simulink model "MicrogridDynamics"  (R2020b)
settings: Solver=ode23t  StartTime=0.0  StopTime=1  RelTol=1e-3
values from neighbouring files (symbols this model uses):
  C = 10e-6    (= 1e-05)    [ControllerDesign.m]
  Frq = 50    [ControllerDesign.m]
  Lg = 1.5e-3    (= 0.0015)    [ControllerDesign.m]
  Li = 3e-3    (= 0.003)    [ControllerDesign.m]
  Ll = 10e-3    (= 0.01)    [ControllerDesign.m]
  Rl = 1    [ControllerDesign.m]
  Rld = 50    [ControllerDesign.m]
  Rld1 = 200    [ControllerDesign.m]
  sw_fr = 10e3    (= 10000)    [ControllerDesign.m]
  Vac = 220    [ControllerDesign.m]
  Vdc = 500    [ControllerDesign.m]
undefined symbols (not defined in the file or in its folder): C_pi, C_pi1
libraries: powerlib x61, powerlib_meascontrol x12, pid_lib x8, eeRmsMeasurement x4, eePowerMeasurement x2
(part 1 of 2)
settings Model: Creator=dipsb  LastModifiedBy=dipsb
settings SolverCC: ZeroCrossAlgorithm=Adaptive
settings DebuggingCC: IgnoredZcDiagnostic=none

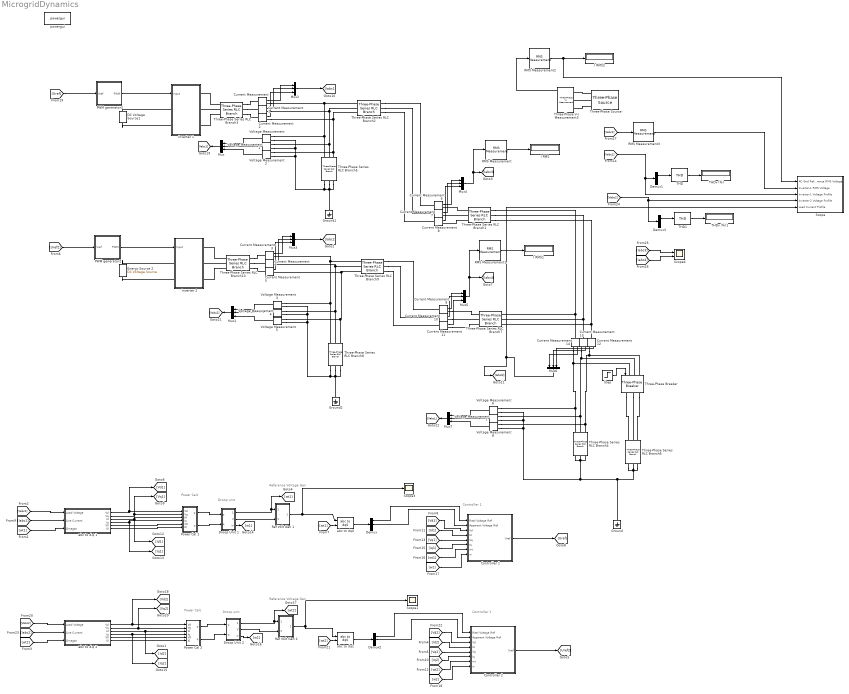
== system MicrogridDynamics ==
  note: Droop unit
  note: Reference Voltage Gen
  note: Reference Voltage Gen
  note: Droop unit
  note: Power Calc
  note: Power Calc
  note: Controller 1
  note: Controller 1
  Controller 1 : Subsystem
  Controller 2 : Subsystem
  Current Measurement{,1..14} (15 alike) : powerlib/Measurements/Current Measurement  PhasorSimulation=off  OutputType=Complex  PSBequivalent=0
  DC Voltage Source1 : powerlib/Electrical Sources/DC Voltage Source  Amplitude=Vdc  Measurements=Voltage
  Demux{,1..3} (4 alike) : Demux  Outputs=3
  Droop Unit 1 : Subsystem
  Droop Unit 2 : Subsystem
  Energy Source 2 : powerlib/Electrical Sources/DC Voltage Source  Amplitude=Vdc  Measurements=Voltage
  Ground : powerlib/Elements/Ground  LConnTagsString=a
  Ground1 : powerlib/Elements/Ground  LConnTagsString=a
  Ground2 : powerlib/Elements/Ground  LConnTagsString=a
  I RMS : Display
  I RMS1 : Display
  I RMS2 : Display
  Inverter 1 : Subsystem
  Inverter 2 : Subsystem
  Mux{,1..7} (8 alike) : Mux  Inputs=3
  PWM generator1 : Subsystem  mask{f=sw_fr}
      mask prompts: f "Frequency (Hz)"
  PWM generator2 : Subsystem  mask{f=sw_fr}
      mask prompts: f "Frequency (Hz)"
  Power Cal 1 : Subsystem
  Power Cal 2 : Subsystem
  RMS Measurement{,1..3} (4 alike) : eeRmsMeasurement/RMS Measurement  LabelModeActiveChoice=Total  F=50  SpecifyHarmonics=off  K=[0 1 2]  Ts=0
      settings: SourceProductBaseCode=PS
  Ref Volt Gen 1 : Subsystem
  Ref Volt Gen 2 : Subsystem
  Scope : Subsystem
  Scope1 : Scope
  Scope3 : Scope
  Scope4 : Scope  NumInputPorts=2
  Step : Step  Time=0.4  SampleTime=0
  THD : powerlib_meascontrol/Measurements/THD  Freq=50  Ts=0
  THD1 : powerlib_meascontrol/Measurements/THD  Freq=50  Ts=0
  THDv (%) : Display
  THDv (%)1 : Display
  Three-Phase Series RLC Branch1 : powerlib/Elements/Three-Phase Series RLC Branch  LConnTagsString=A|B|C  RConnTagsString=A|B|C  BranchType=RL  Resistance=Rl  Inductance=Ll  Capacitance=10e-6  Measurements=None
  Three-Phase Series RLC Branch10 : powerlib/Elements/Three-Phase Series RLC Branch  LConnTagsString=A|B|C  RConnTagsString=A|B|C  BranchType=L  Resistance=1  Inductance=Li  Capacitance=10e-6  Measurements=None
  Three-Phase Series RLC Branch2 : powerlib/Elements/Three-Phase Series RLC Branch  LConnTagsString=A|B|C  RConnTagsString=A|B|C  BranchType=L  Resistance=1  Inductance=Lg  Capacitance=10e-6  Measurements=None
  Three-Phase Series RLC Branch3 : powerlib/Elements/Three-Phase Series RLC Branch  LConnTagsString=A|B|C  RConnTagsString=A|B|C  BranchType=L  Resistance=1  Inductance=Li  Capacitance=10e-6  Measurements=None
  Three-Phase Series RLC Branch4 : powerlib/Elements/Three-Phase Series RLC Branch  LConnTagsString=A|B|C  RConnTagsString=A|B|C  BranchType=R  Resistance=Rld  Inductance=1.5e-3  Capacitance=10e-6  Measurements=None
  Three-Phase Series RLC Branch5 : powerlib/Elements/Three-Phase Series RLC Branch  LConnTagsString=A|B|C  RConnTagsString=A|B|C  BranchType=C  Resistance=1  Inductance=10e-3  Capacitance=C  Measurements=Branch voltages and currents
  Three-Phase Series RLC Branch6 : powerlib/Elements/Three-Phase Series RLC Branch  LConnTagsString=A|B|C  RConnTagsString=A|B|C  BranchType=R  Resistance=Rld1  Inductance=1.5e-3  Capacitance=10e-6  Measurements=None
  Three-Phase Series RLC Branch7 : powerlib/Elements/Three-Phase Series RLC Branch  LConnTagsString=A|B|C  RConnTagsString=A|B|C  BranchType=RL  Resistance=Rl  Inductance=Ll  Capacitance=10e-6  Measurements=None
  Three-Phase Series RLC Branch8 : powerlib/Elements/Three-Phase Series RLC Branch  LConnTagsString=A|B|C  RConnTagsString=A|B|C  BranchType=C  Resistance=1  Inductance=10e-3  Capacitance=C  Measurements=None
  Three-Phase Series RLC Branch9 : powerlib/Elements/Three-Phase Series RLC Branch  LConnTagsString=A|B|C  RConnTagsString=A|B|C  BranchType=L  Resistance=1  Inductance=Lg  Capacitance=10e-6  Measurements=None
  Three-Phase V-I Measurement3 : powerlib/Measurements/Three-Phase V-I Measurement  VoltageMeasurement=phase-to-phase  SetLabelV=off  LabelV=VabcL  Vpu=off  VpuLL=off  CurrentMeasurement=yes  SetLabelI=off  LabelI=Iabc1  Ipu=off  Pbase=100e6  Vbase=500e3  OutputType=Complex  PhasorSimulation=off  PSBequivalent=0
  Three-Phase Breaker : powerlib/Elements/Three-Phase Breaker  InitialState=open  SwitchA=on  SwitchB=on  SwitchC=on  SwitchTimes="[1/60  5/60]"  External=on  BreakerResistance=0.01  SnubberResistance=1e6  SnubberCapacitance=inf  Measurements=None
  Three-Phase Source : powerlib/Electrical Sources/Three-Phase Source  InternalConnection=Yg  VoltagePhases=off  Voltage=Vac  PhaseAngle=0  Voltage_phases=[25e3 25e3 25e3]/sqrt(3)  PhaseAngles_phases=[0 -120 +120]  Frequency=50  NonIdealSource=on  SpecifyImpedance=off  Resistance=0.01  Inductance=16.58e-3  ShortCircuitLevel=100e6  BaseVoltage=Vac  XRratio=7  BusType=swing  Pref=10e3  Qref=0  Prefabc=[10e3, 10e3, 10e3]  Qrefabc=[0, 0, 0]  Qmin=-inf  Qmax=inf
  Voltage Measurement{,1..8} (9 alike) : powerlib/Measurements/Voltage Measurement  PhasorSimulation=off  OutputType=Complex  PSBequivalent=0
  abc to d-q 1 : Subsystem
  abc to d-q 2 : Subsystem
  abc to dq0 : powerlib_meascontrol/Transformations/abc to dq0  Alignment=90 degrees behind phase A axis
  abc to dq1 : powerlib_meascontrol/Transformations/abc to dq0  Alignment=90 degrees behind phase A axis
  powergui : powerlib/powergui  Priority=1  SimulationMode=Discrete  SampleTime=2.5e-6  frequency=60  Iterations=50  frequencyindice=0  Pbase=100e6  ErrMax=1e-4  UnitsV=kV  UnitsW=MW  buscounter=0  FunctionMessages=off  echomessages=off  EnableUseOfTLC=off  CurrentSourceSwitches=off  DisableSnubberDevices=off  DisableRonSwitches=off  DisableVfSwitches=off  DisplayEquations=off  AutomaticDiscreteSolvers=off  SolverType=Tustin/Backward Euler (TBE)  Interpol=off  ExternalGateDelay=off  methode=off  Ts=100  x0status=blocks  SPID=on  SwTol=0  HookPort=off  NonlinearTolerance=1e-4  nMaxIteration=100  ContinueOnMaxIteration=off  RestoreLinks=warning  ResistiveCurrentMeasurement=off  Frange=[0:2:500]  Ylog=off  Xlog=on  ShowGrid=off  save=off  variable=ZData  structure=0  ZoomFFT=off  StartTime=0.0  cycles=1  DisplayStyle=1  fundamental=60  FreqAxis=off  MaxFrequency=1000  frequencyindicesteady=1  RmsSteady=1  display=off
  wires:
  THD/1 -> THDv (%)/1
  Demux1/1 -> THD/1
  [Uref] -> PWM generator1/1(Vref)
  [Vabc1] -> Scope/3(Inverter-1 Voltage Profile), Demux1/1
  Mux3/1 -> [Iabc2]
  PWM generator1/1(PWM) -> Inverter 1/1(Input)
  Controller 1/1(Uref) -> [Uref]
  [Iabc1] -> abc to d-q 1/2(Line Current)
  [Vabc1] -> abc to d-q 1/1(Load Voltage)
  [wt1] -> abc to d-q 1/3(Omegat)
  [Uref2] -> PWM generator2/1(Vref)
  abc to d-q 1/1(Vd) -> [Vd1], Power Cal 1/1(Vd)
  abc to d-q 1/2(Vq) -> Power Cal 1/2(Vq), [Vq1]
  abc to d-q 1/3(Id) -> [Id1], Power Cal 1/3(Id)
  abc to d-q 1/4(Iq) -> [Iq1], Power Cal 1/4(Iq)
  Droop Unit 1/1(thetat) -> Ref Volt Gen 1/1(theta), [wt1]
  Droop Unit 1/2(V) -> Ref Volt Gen 1/2(V)
  Ref Volt Gen 1/1(Vabc) -> abc to dq0/1, Scope3/1
  abc to dq0/1 -> Demux/1
  Demux/1 -> Controller 1/1(Real Voltage Ref)
  Demux/2 -> Controller 1/2(Apparent Voltage Ref)
  RMS Measurement/1 -> I RMS/1
  Step/1 -> Three-Phase Breaker/1
  Three-Phase V-I Measurement3/1 -> RMS Measurement2/1
  RMS Measurement2/1 -> Scope/1("AC Grid Reference RMS Voltage  "), I RMS2/1
  PWM generator2/1(PWM) -> Inverter 2/1(Input)
  Mux2/1 -> [Iabc1]
  Mux6/1 -> Scope/5(Load Current Profile), [Iabcld]
  Mux5/1 -> RMS Measurement1/1, [Iabc4]
  Mux4/1 -> RMS Measurement/1, [Iabc3]
  RMS Measurement1/1 -> I RMS1/1
  [wt1] -> abc to dq0/2
  Droop Unit 1/3(w) -> [w1]
  [Vd1] -> Controller 1/3(Vd)
  [Id1] -> Controller 1/4(Id)
  [Vq1] -> Controller 1/5(Vq)
  [Iq1] -> Controller 1/6(Iq)
  [wt1] -> Controller 1/7(wt)
  [w1] -> Controller 1/8(w)
  [wt2] -> Controller 2/7(wt)
  [Iq2] -> Controller 2/6(Iq)
  Droop Unit 2/2(V) -> Ref Volt Gen 2/2(V)
  Demux2/2 -> Controller 2/2(Apparent Voltage Ref)
  Droop Unit 2/3(w) -> [w2]
  Ref Volt Gen 2/1(Vabc) -> abc to dq1/1, Scope1/1
  [Iabc2] -> abc to d-q 2/2(Line Current)
  Demux2/1 -> Controller 2/1(Real Voltage Ref)
  abc to dq1/1 -> Demux2/1
  abc to d-q 2/4(Iq) -> [Iq2], Power Cal 2/4(Iq)
  [Id2] -> Controller 2/4(Id)
  abc to d-q 2/1(Vd) -> [Vd2], Power Cal 2/1(Vd)
  [Vd2] -> Controller 2/3(Vd)
  [Vabc2] -> abc to d-q 2/1(Load Voltage)
  Controller 2/1(Uref) -> [Uref2]
  [wt2] -> abc to dq1/2
  [Vq2] -> Controller 2/5(Vq)
  [wt2] -> abc to d-q 2/3(Omegat)
  [w2] -> Controller 2/8(w)
  Droop Unit 2/1(thetat) -> Ref Volt Gen 2/1(theta), [wt2]
  THD1/1 -> THDv (%)1/1
  Demux3/1 -> THD1/1
  [Vabc2] -> Scope/4(Inverter-2 Voltage Profile), Demux3/1
  [Iabc3] -> Scope4/1
  [Iabc4] -> Scope4/2
  [Vabc1] -> RMS Measurement3/1
  Voltage Measurement2/1 -> Mux/3
  Voltage Measurement1/1 -> Mux/2
  Voltage Measurement/1 -> Mux/1
  Mux/1 -> [Vabc1]
  Voltage Measurement5/1 -> Mux1/3
  Mux1/1 -> [Vabc2]
  Voltage Measurement3/1 -> Mux1/1
  Voltage Measurement4/1 -> Mux1/2
  Current Measurement/1 -> Mux2/1
  Current Measurement1/1 -> Mux2/2
  Current Measurement2/1 -> Mux2/3
  Current Measurement3/1 -> Mux3/1
  Current Measurement4/1 -> Mux3/2
  Current Measurement5/1 -> Mux3/3
  Current Measurement6/1 -> Mux4/1
  Current Measurement8/1 -> Mux4/3
  Current Measurement7/1 -> Mux4/2
  Current Measurement9/1 -> Mux5/1
  Current Measurement11/1 -> Mux5/3
  Current Measurement10/1 -> Mux5/2
  Current Measurement14/1 -> Mux6/1
  Current Measurement13/1 -> Mux6/2
  Current Measurement12/1 -> Mux6/3
  Voltage Measurement6/1 -> Mux7/1
  Voltage Measurement7/1 -> Mux7/2
  Mux7/1 -> [VabcL]
  Voltage Measurement8/1 -> Mux7/3
  Power Cal 1/1(p) -> Droop Unit 1/1(p)
  Power Cal 1/2(q) -> Droop Unit 1/2(q)
  Power Cal 2/1(p) -> Droop Unit 2/1(p)
  Power Cal 2/2(q) -> Droop Unit 2/2(q)
  RMS Measurement3/1 -> Scope/2("Inverter-1 RMS Voltage  ")
  abc to d-q 1/5(V0) -> Power Cal 1/5(V0)
  abc to d-q 1/6(I0) -> Power Cal 1/6(I0)
  abc to d-q 2/2(Vq) -> [Vq2], Power Cal 2/2(Vq)
  abc to d-q 2/3(Id) -> Power Cal 2/3(Id), [Id2]
  abc to d-q 2/5(V0) -> Power Cal 2/5(V0)
  abc to d-q 2/6(I0) -> Power Cal 2/6(I0)
  connections:
  DC Voltage Source1/RConn1 -- Inverter 1/LConn1
  DC Voltage Source1/LConn1 -- Inverter 1/LConn2
  Three-Phase Series RLC Branch3/LConn1 -- Inverter 1/RConn1
  Three-Phase Series RLC Branch3/LConn2 -- Inverter 1/RConn2
  Three-Phase Series RLC Branch3/LConn3 -- Inverter 1/RConn3
  Three-Phase Series RLC Branch7/RConn1 -- Three-Phase Series RLC Branch1/RConn1 -- Current Measurement14/LConn1
  Ground1/LConn1 -- Voltage Measurement2/LConn2 -- Voltage Measurement1/LConn2 -- Voltage Measurement/LConn2 -- Three-Phase Series RLC Branch5/RConn1 -- Three-Phase Series RLC Branch5/RConn3 -- Three-Phase Series RLC Branch5/RConn2
  Voltage Measurement1/LConn1 -- Current Measurement1/RConn1 -- Three-Phase Series RLC Branch2/LConn2 -- Three-Phase Series RLC Branch5/LConn2
  Voltage Measurement2/LConn1 -- Three-Phase Series RLC Branch2/LConn3 -- Current Measurement2/RConn1 -- Three-Phase Series RLC Branch5/LConn3
  Energy Source 2/LConn1 -- Inverter 2/LConn2
  Three-Phase Series RLC Branch10/LConn1 -- Inverter 2/RConn1
  Three-Phase Series RLC Branch10/LConn2 -- Inverter 2/RConn2
  Energy Source 2/RConn1 -- Inverter 2/LConn1
  Voltage Measurement5/LConn1 -- Three-Phase Series RLC Branch9/LConn3 -- Current Measurement5/RConn1 -- Three-Phase Series RLC Branch8/LConn3
  Voltage Measurement6/LConn2 -- Voltage Measurement7/LConn2 -- Voltage Measurement8/LConn2 -- Ground/LConn1 -- Three-Phase Series RLC Branch6/RConn1 -- Three-Phase Series RLC Branch6/RConn2 -- Three-Phase Series RLC Branch6/RConn3 -- Three-Phase Series RLC Branch4/RConn1 -- Three-Phase Series RLC Branch4/RConn2 -- Three-Phase Series RLC Branch4/RConn3
  Three-Phase Source/RConn1 -- Three-Phase V-I Measurement3/LConn1
  Three-Phase Source/RConn2 -- Three-Phase V-I Measurement3/LConn2
  Three-Phase Source/RConn3 -- Three-Phase V-I Measurement3/LConn3
  Voltage Measurement3/LConn1 -- Three-Phase Series RLC Branch8/LConn1 -- Current Measurement3/RConn1 -- Three-Phase Series RLC Branch9/LConn1
  Three-Phase Series RLC Branch8/LConn2 -- Voltage Measurement4/LConn1 -- Current Measurement4/RConn1 -- Three-Phase Series RLC Branch9/LConn2
  Current Measurement11/RConn1 -- Three-Phase Series RLC Branch7/LConn3
  Current Measurement9/RConn1 -- Three-Phase Series RLC Branch7/LConn1
  Current Measurement10/RConn1 -- Three-Phase Series RLC Branch7/LConn2
  Three-Phase Series RLC Branch3/RConn1 -- Current Measurement/LConn1
  Three-Phase Series RLC Branch3/RConn2 -- Current Measurement1/LConn1
  Three-Phase Series RLC Branch3/RConn3 -- Current Measurement2/LConn1
  Three-Phase Series RLC Branch10/LConn3 -- Inverter 2/RConn3
  Three-Phase Series RLC Branch7/RConn2 -- Three-Phase Series RLC Branch1/RConn2 -- Current Measurement13/LConn1
  Three-Phase Series RLC Branch7/RConn3 -- Three-Phase Series RLC Branch1/RConn3 -- Current Measurement12/LConn1
  Voltage Measurement/LConn1 -- Three-Phase Series RLC Branch5/LConn1 -- Current Measurement/RConn1 -- Three-Phase Series RLC Branch2/LConn1
  Three-Phase Series RLC Branch10/RConn2 -- Current Measurement4/LConn1
  Three-Phase Series RLC Branch10/RConn1 -- Current Measurement3/LConn1
  Three-Phase Series RLC Branch10/RConn3 -- Current Measurement5/LConn1
  Voltage Measurement3/LConn2 -- Voltage Measurement5/LConn2 -- Ground2/LConn1 -- Three-Phase Series RLC Branch8/RConn3 -- Three-Phase Series RLC Branch8/RConn2 -- Three-Phase Series RLC Branch8/RConn1 -- Voltage Measurement4/LConn2
  Three-Phase Series RLC Branch1/LConn2 -- Current Measurement7/RConn1
  Three-Phase Series RLC Branch1/LConn1 -- Current Measurement6/RConn1
  Three-Phase Series RLC Branch1/LConn3 -- Current Measurement8/RConn1
  Current Measurement14/RConn1 -- Three-Phase Breaker/LConn1 -- Voltage Measurement6/LConn1 -- Three-Phase Series RLC Branch4/LConn1
  Three-Phase Breaker/LConn2 -- Current Measurement13/RConn1 -- Voltage Measurement7/LConn1 -- Three-Phase Series RLC Branch4/LConn2
  Three-Phase Breaker/LConn3 -- Current Measurement12/RConn1 -- Voltage Measurement8/LConn1 -- Three-Phase Series RLC Branch4/LConn3
  Three-Phase Breaker/RConn1 -- Three-Phase Series RLC Branch6/LConn1
  Three-Phase Breaker/RConn2 -- Three-Phase Series RLC Branch6/LConn2
  Three-Phase Breaker/RConn3 -- Three-Phase Series RLC Branch6/LConn3
  Three-Phase Series RLC Branch2/RConn1 -- Current Measurement6/LConn1
  Three-Phase Series RLC Branch2/RConn2 -- Current Measurement7/LConn1
  Three-Phase Series RLC Branch2/RConn3 -- Current Measurement8/LConn1
  Three-Phase Series RLC Branch9/RConn1 -- Current Measurement9/LConn1
  Three-Phase Series RLC Branch9/RConn2 -- Current Measurement10/LConn1
  Three-Phase Series RLC Branch9/RConn3 -- Current Measurement11/LConn1

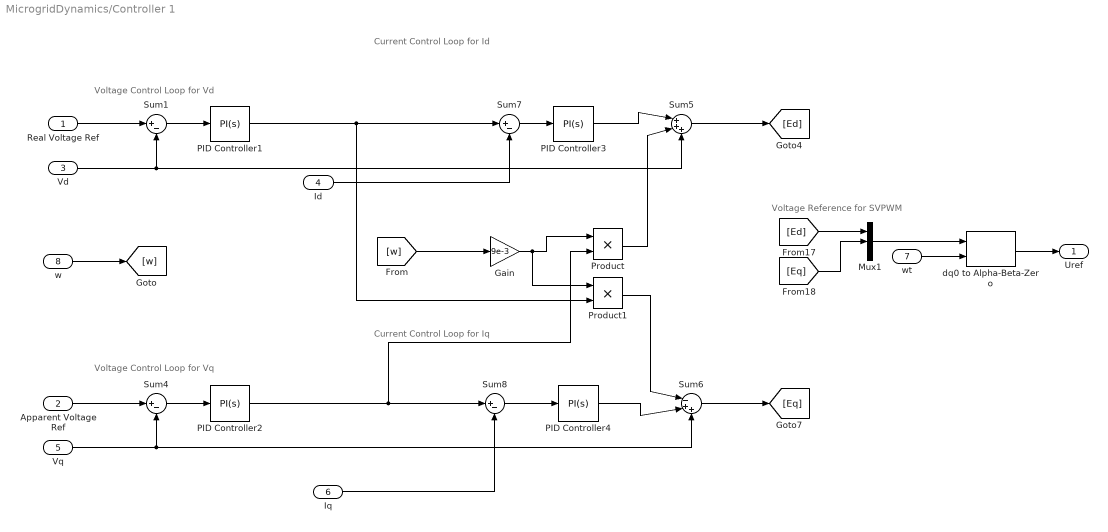
== system MicrogridDynamics/Controller 1 ==
  note: Current Control Loop for Iq
  note: Current Control Loop for Id
  note: Voltage Control Loop for Vd
  note: Voltage Control Loop for Vq
  note: Voltage Reference for SVPWM
  Real Voltage Ref : Inport
  Apparent Voltage Ref : Inport  Port=2
  Vd : Inport  Port=3
  Id : Inport  Port=4
  Vq : Inport  Port=5
  Iq : Inport  Port=6
  wt : Inport  Port=7
  w : Inport  Port=8
  Gain : Gain  Gain=9e-3
  Mux1 : Mux  Inputs=3
  PID Controller1 : pid_lib/PID Controller  Controller=PI  Form=Parallel  TimeDomain=Continuous-time  UseExternalTs=off  SampleTime=-1  IntegratorMethod=Forward Euler  FilterMethod=Forward Euler  ControllerParametersSource=internal  P=(C_pi1.Kp)  I=(C_pi1.Ki)  D=0  UseFilter=on  N=100  TunerSelectOption=Transfer Function Based (PID Tuner App)  InitialConditionSource=internal  InitialConditionForIntegrator=0  InitialConditionForFilter=0  DifferentiatorICPrevScaledInput=0  ExternalReset=none  TrackingMode=off  Kt=1  LimitOutput=off  SatLimitsSource=internal  UpperSaturationLimit=0.95  LowerSaturationLimit=0.275  LinearizeAsGain=on  AntiWindupMode=none  Kb=1  POutMin=[]  POutMax=[]  IOutMin=[]  IOutMax=[]  DOutMin=[]  DOutMax=[]  NOutMin=[]  NOutMax=[]  SumOutMin=[]  SumOutMax=[]  SaturationOutMin=[]  SaturationOutMax=[]  PParamMin=[]  PParamMax=[]  IParamMin=[]  IParamMax=[]  DParamMin=[]  DParamMax=[]  NParamMin=[]  NParamMax=[]  KbParamMin=[]  KbParamMax=[]  KtParamMin=[]  KtParamMax=[]  KbOutMin=[]  KbOutMax=[]  KtOutMin=[]  KtOutMax=[]  IntegratorOutMin=[]  IntegratorOutMax=[]  FilterOutMin=[]  FilterOutMax=[]  SumI1OutMin=[]  SumI1OutMax=[]  SumI2OutMin=[]  SumI2OutMax=[]  SumI3OutMin=[]  SumI3OutMax=[]  SumI4OutMin=[]  SumI4OutMax=[]  SumDOutMin=[]  SumDOutMax=[]  DifferentiatorOutMin=[]  DifferentiatorOutMax=[]  FilterDiffOutCoefMin=[]  FilterDiffOutCoefMax=[]  ReciprocalOutMin=[]  ReciprocalOutMax=[]  SumDenOutMin=[]  SumDenOutMax=[]  SumNumOutMin=[]  SumNumOutMax=[]  DivideOutMin=[]  DivideOutMax=[]  UdiffTsProdOutMin=[]  UdiffTsProdOutMax=[]  NTsProdOutMin=[]  NTsProdOutMax=[]  UintegralTsProdOutMin=[]  UintegralTsProdOutMax=[]  UngainTsProdOutMin=[]  UngainTsProdOutMax=[]  IntegratorContinuousStateAttributes=''  IntegratorStateMustResolveToSignalObject=off  IntegratorRTWStateStorageClass=Auto  FilterContinuousStateAttributes=''  FilterStateMustResolveToSignalObject=off  FilterRTWStateStorageClass=Auto  ParallelPVariant=InternalParameters  IdealPVariant=Disabled  IVariant=InternalParameters  DVariant=Disabled  IntegratorVariant=Continuous  SatVariant=Disabled  AWVariant=Passthrough  PCopyVariant=Disabled  TRVariant=Disabled  FdbkBlocksVariant=Forward  IdealPFdbkVariant=Disabled  SatFdbkVariant=Disabled  DerivativeFilterVariant=Disabled  NVariant=Disabled  NCopyVariant=Disabled_SignalSpec  FilterICVariant=Disabled  IntegratorICVariant=InternalICs  ExternalResetVariant=Disabled  TRSumVariant=Passthrough  SumFdbkVariant=Disabled  SumVariant=Sum_PI  TsampFilterVariant=InternalTs  TsampNgainVariant=Passthrough  TsampIntegralVariant=Passthrough  ExternalSaturationOutDataTypeStr=Inherit: Same as second input
  PID Controller2 : pid_lib/PID Controller  Controller=PI  Form=Parallel  TimeDomain=Continuous-time  UseExternalTs=off  SampleTime=-1  IntegratorMethod=Forward Euler  FilterMethod=Forward Euler  ControllerParametersSource=internal  P=C_pi1.Kp  I=C_pi1.Ki  D=0  UseFilter=on  N=100  TunerSelectOption=Transfer Function Based (PID Tuner App)  InitialConditionSource=internal  InitialConditionForIntegrator=0  InitialConditionForFilter=0  DifferentiatorICPrevScaledInput=0  ExternalReset=none  TrackingMode=off  Kt=1  LimitOutput=off  SatLimitsSource=internal  UpperSaturationLimit=0.95  LowerSaturationLimit=0.275  LinearizeAsGain=on  AntiWindupMode=none  Kb=1  POutMin=[]  POutMax=[]  IOutMin=[]  IOutMax=[]  DOutMin=[]  DOutMax=[]  NOutMin=[]  NOutMax=[]  SumOutMin=[]  SumOutMax=[]  SaturationOutMin=[]  SaturationOutMax=[]  PParamMin=[]  PParamMax=[]  IParamMin=[]  IParamMax=[]  DParamMin=[]  DParamMax=[]  NParamMin=[]  NParamMax=[]  KbParamMin=[]  KbParamMax=[]  KtParamMin=[]  KtParamMax=[]  KbOutMin=[]  KbOutMax=[]  KtOutMin=[]  KtOutMax=[]  IntegratorOutMin=[]  IntegratorOutMax=[]  FilterOutMin=[]  FilterOutMax=[]  SumI1OutMin=[]  SumI1OutMax=[]  SumI2OutMin=[]  SumI2OutMax=[]  SumI3OutMin=[]  SumI3OutMax=[]  SumI4OutMin=[]  SumI4OutMax=[]  SumDOutMin=[]  SumDOutMax=[]  DifferentiatorOutMin=[]  DifferentiatorOutMax=[]  FilterDiffOutCoefMin=[]  FilterDiffOutCoefMax=[]  ReciprocalOutMin=[]  ReciprocalOutMax=[]  SumDenOutMin=[]  SumDenOutMax=[]  SumNumOutMin=[]  SumNumOutMax=[]  DivideOutMin=[]  DivideOutMax=[]  UdiffTsProdOutMin=[]  UdiffTsProdOutMax=[]  NTsProdOutMin=[]  NTsProdOutMax=[]  UintegralTsProdOutMin=[]  UintegralTsProdOutMax=[]  UngainTsProdOutMin=[]  UngainTsProdOutMax=[]  IntegratorContinuousStateAttributes=''  IntegratorStateMustResolveToSignalObject=off  IntegratorRTWStateStorageClass=Auto  FilterContinuousStateAttributes=''  FilterStateMustResolveToSignalObject=off  FilterRTWStateStorageClass=Auto  ParallelPVariant=InternalParameters  IdealPVariant=Disabled  IVariant=InternalParameters  DVariant=Disabled  IntegratorVariant=Continuous  SatVariant=Disabled  AWVariant=Passthrough  PCopyVariant=Disabled  TRVariant=Disabled  FdbkBlocksVariant=Forward  IdealPFdbkVariant=Disabled  SatFdbkVariant=Disabled  DerivativeFilterVariant=Disabled  NVariant=Disabled  NCopyVariant=Disabled_SignalSpec  FilterICVariant=Disabled  IntegratorICVariant=InternalICs  ExternalResetVariant=Disabled  TRSumVariant=Passthrough  SumFdbkVariant=Disabled  SumVariant=Sum_PI  TsampFilterVariant=InternalTs  TsampNgainVariant=Passthrough  TsampIntegralVariant=Passthrough  ExternalSaturationOutDataTypeStr=Inherit: Same as second input
  PID Controller3 : pid_lib/PID Controller  Controller=PI  Form=Parallel  TimeDomain=Continuous-time  UseExternalTs=off  SampleTime=-1  IntegratorMethod=Forward Euler  FilterMethod=Forward Euler  ControllerParametersSource=internal  P=C_pi.Kp  I=C_pi.Ki  D=0  UseFilter=on  N=100  TunerSelectOption=Frequency Response Based  InitialConditionSource=internal  InitialConditionForIntegrator=0  InitialConditionForFilter=0  DifferentiatorICPrevScaledInput=0  ExternalReset=none  TrackingMode=off  Kt=1  LimitOutput=off  SatLimitsSource=internal  UpperSaturationLimit=0.95  LowerSaturationLimit=0.275  LinearizeAsGain=on  AntiWindupMode=none  Kb=1  POutMin=[]  POutMax=[]  IOutMin=[]  IOutMax=[]  DOutMin=[]  DOutMax=[]  NOutMin=[]  NOutMax=[]  SumOutMin=[]  SumOutMax=[]  SaturationOutMin=[]  SaturationOutMax=[]  PParamMin=[]  PParamMax=[]  IParamMin=[]  IParamMax=[]  DParamMin=[]  DParamMax=[]  NParamMin=[]  NParamMax=[]  KbParamMin=[]  KbParamMax=[]  KtParamMin=[]  KtParamMax=[]  KbOutMin=[]  KbOutMax=[]  KtOutMin=[]  KtOutMax=[]  IntegratorOutMin=[]  IntegratorOutMax=[]  FilterOutMin=[]  FilterOutMax=[]  SumI1OutMin=[]  SumI1OutMax=[]  SumI2OutMin=[]  SumI2OutMax=[]  SumI3OutMin=[]  SumI3OutMax=[]  SumI4OutMin=[]  SumI4OutMax=[]  SumDOutMin=[]  SumDOutMax=[]  DifferentiatorOutMin=[]  DifferentiatorOutMax=[]  FilterDiffOutCoefMin=[]  FilterDiffOutCoefMax=[]  ReciprocalOutMin=[]  ReciprocalOutMax=[]  SumDenOutMin=[]  SumDenOutMax=[]  SumNumOutMin=[]  SumNumOutMax=[]  DivideOutMin=[]  DivideOutMax=[]  UdiffTsProdOutMin=[]  UdiffTsProdOutMax=[]  NTsProdOutMin=[]  NTsProdOutMax=[]  UintegralTsProdOutMin=[]  UintegralTsProdOutMax=[]  UngainTsProdOutMin=[]  UngainTsProdOutMax=[]  IntegratorContinuousStateAttributes=''  IntegratorStateMustResolveToSignalObject=off  IntegratorRTWStateStorageClass=Auto  FilterContinuousStateAttributes=''  FilterStateMustResolveToSignalObject=off  FilterRTWStateStorageClass=Auto  ParallelPVariant=InternalParameters  IdealPVariant=Disabled  IVariant=InternalParameters  DVariant=Disabled  IntegratorVariant=Continuous  SatVariant=Disabled  AWVariant=Passthrough  PCopyVariant=Disabled  TRVariant=Disabled  FdbkBlocksVariant=Forward  IdealPFdbkVariant=Disabled  SatFdbkVariant=Disabled  DerivativeFilterVariant=Disabled  NVariant=Disabled  NCopyVariant=Disabled_SignalSpec  FilterICVariant=Disabled  IntegratorICVariant=InternalICs  ExternalResetVariant=Disabled  TRSumVariant=Passthrough  SumFdbkVariant=Disabled  SumVariant=Sum_PI  TsampFilterVariant=InternalTs  TsampNgainVariant=Passthrough  TsampIntegralVariant=Passthrough  ExternalSaturationOutDataTypeStr=Inherit: Same as second input
  PID Controller4 : pid_lib/PID Controller  Controller=PI  Form=Parallel  TimeDomain=Continuous-time  UseExternalTs=off  SampleTime=-1  IntegratorMethod=Forward Euler  FilterMethod=Forward Euler  ControllerParametersSource=internal  P=C_pi.Kp  I=C_pi.Ki  D=0  UseFilter=on  N=100  TunerSelectOption=Frequency Response Based  InitialConditionSource=internal  InitialConditionForIntegrator=0  InitialConditionForFilter=0  DifferentiatorICPrevScaledInput=0  ExternalReset=none  TrackingMode=off  Kt=1  LimitOutput=off  SatLimitsSource=internal  UpperSaturationLimit=0.95  LowerSaturationLimit=0.275  LinearizeAsGain=on  AntiWindupMode=none  Kb=1  POutMin=[]  POutMax=[]  IOutMin=[]  IOutMax=[]  DOutMin=[]  DOutMax=[]  NOutMin=[]  NOutMax=[]  SumOutMin=[]  SumOutMax=[]  SaturationOutMin=[]  SaturationOutMax=[]  PParamMin=[]  PParamMax=[]  IParamMin=[]  IParamMax=[]  DParamMin=[]  DParamMax=[]  NParamMin=[]  NParamMax=[]  KbParamMin=[]  KbParamMax=[]  KtParamMin=[]  KtParamMax=[]  KbOutMin=[]  KbOutMax=[]  KtOutMin=[]  KtOutMax=[]  IntegratorOutMin=[]  IntegratorOutMax=[]  FilterOutMin=[]  FilterOutMax=[]  SumI1OutMin=[]  SumI1OutMax=[]  SumI2OutMin=[]  SumI2OutMax=[]  SumI3OutMin=[]  SumI3OutMax=[]  SumI4OutMin=[]  SumI4OutMax=[]  SumDOutMin=[]  SumDOutMax=[]  DifferentiatorOutMin=[]  DifferentiatorOutMax=[]  FilterDiffOutCoefMin=[]  FilterDiffOutCoefMax=[]  ReciprocalOutMin=[]  ReciprocalOutMax=[]  SumDenOutMin=[]  SumDenOutMax=[]  SumNumOutMin=[]  SumNumOutMax=[]  DivideOutMin=[]  DivideOutMax=[]  UdiffTsProdOutMin=[]  UdiffTsProdOutMax=[]  NTsProdOutMin=[]  NTsProdOutMax=[]  UintegralTsProdOutMin=[]  UintegralTsProdOutMax=[]  UngainTsProdOutMin=[]  UngainTsProdOutMax=[]  IntegratorContinuousStateAttributes=''  IntegratorStateMustResolveToSignalObject=off  IntegratorRTWStateStorageClass=Auto  FilterContinuousStateAttributes=''  FilterStateMustResolveToSignalObject=off  FilterRTWStateStorageClass=Auto  ParallelPVariant=InternalParameters  IdealPVariant=Disabled  IVariant=InternalParameters  DVariant=Disabled  IntegratorVariant=Continuous  SatVariant=Disabled  AWVariant=Passthrough  PCopyVariant=Disabled  TRVariant=Disabled  FdbkBlocksVariant=Forward  IdealPFdbkVariant=Disabled  SatFdbkVariant=Disabled  DerivativeFilterVariant=Disabled  NVariant=Disabled  NCopyVariant=Disabled_SignalSpec  FilterICVariant=Disabled  IntegratorICVariant=InternalICs  ExternalResetVariant=Disabled  TRSumVariant=Passthrough  SumFdbkVariant=Disabled  SumVariant=Sum_PI  TsampFilterVariant=InternalTs  TsampNgainVariant=Passthrough  TsampIntegralVariant=Passthrough  ExternalSaturationOutDataTypeStr=Inherit: Same as second input
  Product : Product
  Product1 : Product
  Sum{1,4,7..8} (4 alike) : Sum  Inputs=|+-
  Sum5 : Sum  Inputs=|+++
  Sum6 : Sum  Inputs=|-++
  dq0 to Alpha-Beta-Zero : powerlib_meascontrol/Transformations/dq0 to Alpha-Beta-Zero  Alignment=90 degrees behind phase A axis
      settings: SourceProductBaseCode=PS
  Uref : Outport
  wires:
  Sum1/1 -> PID Controller1/1
  Vq/1 -> Sum6/3, Sum4/2
  Mux1/1 -> dq0 to Alpha-Beta-Zero/1
  [Ed] -> Mux1/1
  Sum4/1 -> PID Controller2/1
  Vd/1 -> Sum5/3, Sum1/2
  Apparent Voltage Ref/1 -> Sum4/1
  [Eq] -> Mux1/2
  Real Voltage Ref/1 -> Sum1/1
  PID Controller1/1 -> Product1/2, Sum7/1
  PID Controller2/1 -> Product/2, Sum8/1
  PID Controller4/1 -> Sum6/2
  wt/1 -> dq0 to Alpha-Beta-Zero/2
  dq0 to Alpha-Beta-Zero/1 -> Uref/1
  [w] -> Gain/1
  PID Controller3/1 -> Sum5/1
  Sum5/1 -> [Ed]
  Product/1 -> Sum5/2
  Sum6/1 -> [Eq]
  Gain/1 -> Product1/1, Product/1
  Product1/1 -> Sum6/1
  w/1 -> [w]
  Sum7/1 -> PID Controller3/1
  Id/1 -> Sum7/2
  Sum8/1 -> PID Controller4/1
  Iq/1 -> Sum8/2

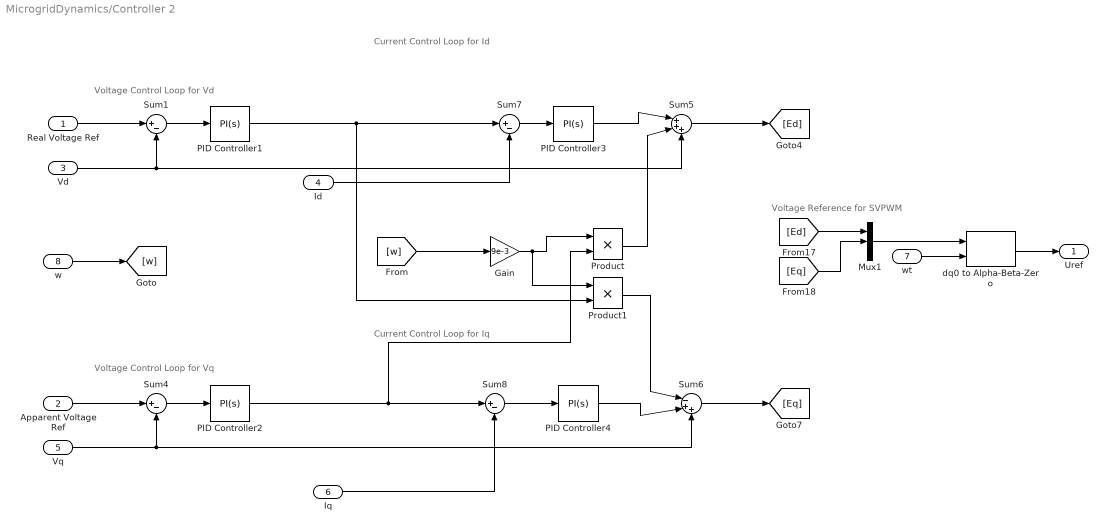
== system MicrogridDynamics/Controller 2 ==
  note: Current Control Loop for Iq
  note: Current Control Loop for Id
  note: Voltage Control Loop for Vd
  note: Voltage Control Loop for Vq
  note: Voltage Reference for SVPWM
  Real Voltage Ref : Inport
  Apparent Voltage Ref : Inport  Port=2
  Vd : Inport  Port=3
  Id : Inport  Port=4
  Vq : Inport  Port=5
  Iq : Inport  Port=6
  wt : Inport  Port=7
  w : Inport  Port=8
  Gain : Gain  Gain=9e-3
  Mux1 : Mux  Inputs=3
  PID Controller1 : pid_lib/PID Controller  Controller=PI  Form=Parallel  TimeDomain=Continuous-time  UseExternalTs=off  SampleTime=-1  IntegratorMethod=Forward Euler  FilterMethod=Forward Euler  ControllerParametersSource=internal  P=C_pi1.Kp  I=C_pi1.Ki  D=0  UseFilter=on  N=100  TunerSelectOption=Transfer Function Based (PID Tuner App)  InitialConditionSource=internal  InitialConditionForIntegrator=0  InitialConditionForFilter=0  DifferentiatorICPrevScaledInput=0  ExternalReset=none  TrackingMode=off  Kt=1  LimitOutput=off  SatLimitsSource=internal  UpperSaturationLimit=0.95  LowerSaturationLimit=0.275  LinearizeAsGain=on  AntiWindupMode=none  Kb=1  POutMin=[]  POutMax=[]  IOutMin=[]  IOutMax=[]  DOutMin=[]  DOutMax=[]  NOutMin=[]  NOutMax=[]  SumOutMin=[]  SumOutMax=[]  SaturationOutMin=[]  SaturationOutMax=[]  PParamMin=[]  PParamMax=[]  IParamMin=[]  IParamMax=[]  DParamMin=[]  DParamMax=[]  NParamMin=[]  NParamMax=[]  KbParamMin=[]  KbParamMax=[]  KtParamMin=[]  KtParamMax=[]  KbOutMin=[]  KbOutMax=[]  KtOutMin=[]  KtOutMax=[]  IntegratorOutMin=[]  IntegratorOutMax=[]  FilterOutMin=[]  FilterOutMax=[]  SumI1OutMin=[]  SumI1OutMax=[]  SumI2OutMin=[]  SumI2OutMax=[]  SumI3OutMin=[]  SumI3OutMax=[]  SumI4OutMin=[]  SumI4OutMax=[]  SumDOutMin=[]  SumDOutMax=[]  DifferentiatorOutMin=[]  DifferentiatorOutMax=[]  FilterDiffOutCoefMin=[]  FilterDiffOutCoefMax=[]  ReciprocalOutMin=[]  ReciprocalOutMax=[]  SumDenOutMin=[]  SumDenOutMax=[]  SumNumOutMin=[]  SumNumOutMax=[]  DivideOutMin=[]  DivideOutMax=[]  UdiffTsProdOutMin=[]  UdiffTsProdOutMax=[]  NTsProdOutMin=[]  NTsProdOutMax=[]  UintegralTsProdOutMin=[]  UintegralTsProdOutMax=[]  UngainTsProdOutMin=[]  UngainTsProdOutMax=[]  IntegratorContinuousStateAttributes=''  IntegratorStateMustResolveToSignalObject=off  IntegratorRTWStateStorageClass=Auto  FilterContinuousStateAttributes=''  FilterStateMustResolveToSignalObject=off  FilterRTWStateStorageClass=Auto  ParallelPVariant=InternalParameters  IdealPVariant=Disabled  IVariant=InternalParameters  DVariant=Disabled  IntegratorVariant=Continuous  SatVariant=Disabled  AWVariant=Passthrough  PCopyVariant=Disabled  TRVariant=Disabled  FdbkBlocksVariant=Forward  IdealPFdbkVariant=Disabled  SatFdbkVariant=Disabled  DerivativeFilterVariant=Disabled  NVariant=Disabled  NCopyVariant=Disabled_SignalSpec  FilterICVariant=Disabled  IntegratorICVariant=InternalICs  ExternalResetVariant=Disabled  TRSumVariant=Passthrough  SumFdbkVariant=Disabled  SumVariant=Sum_PI  TsampFilterVariant=InternalTs  TsampNgainVariant=Passthrough  TsampIntegralVariant=Passthrough  ExternalSaturationOutDataTypeStr=Inherit: Same as second input
  PID Controller2 : pid_lib/PID Controller  Controller=PI  Form=Parallel  TimeDomain=Continuous-time  UseExternalTs=off  SampleTime=-1  IntegratorMethod=Forward Euler  FilterMethod=Forward Euler  ControllerParametersSource=internal  P=C_pi1.Kp  I=C_pi1.Ki  D=0  UseFilter=on  N=100  TunerSelectOption=Transfer Function Based (PID Tuner App)  InitialConditionSource=internal  InitialConditionForIntegrator=0  InitialConditionForFilter=0  DifferentiatorICPrevScaledInput=0  ExternalReset=none  TrackingMode=off  Kt=1  LimitOutput=off  SatLimitsSource=internal  UpperSaturationLimit=0.95  LowerSaturationLimit=0.275  LinearizeAsGain=on  AntiWindupMode=none  Kb=1  POutMin=[]  POutMax=[]  IOutMin=[]  IOutMax=[]  DOutMin=[]  DOutMax=[]  NOutMin=[]  NOutMax=[]  SumOutMin=[]  SumOutMax=[]  SaturationOutMin=[]  SaturationOutMax=[]  PParamMin=[]  PParamMax=[]  IParamMin=[]  IParamMax=[]  DParamMin=[]  DParamMax=[]  NParamMin=[]  NParamMax=[]  KbParamMin=[]  KbParamMax=[]  KtParamMin=[]  KtParamMax=[]  KbOutMin=[]  KbOutMax=[]  KtOutMin=[]  KtOutMax=[]  IntegratorOutMin=[]  IntegratorOutMax=[]  FilterOutMin=[]  FilterOutMax=[]  SumI1OutMin=[]  SumI1OutMax=[]  SumI2OutMin=[]  SumI2OutMax=[]  SumI3OutMin=[]  SumI3OutMax=[]  SumI4OutMin=[]  SumI4OutMax=[]  SumDOutMin=[]  SumDOutMax=[]  DifferentiatorOutMin=[]  DifferentiatorOutMax=[]  FilterDiffOutCoefMin=[]  FilterDiffOutCoefMax=[]  ReciprocalOutMin=[]  ReciprocalOutMax=[]  SumDenOutMin=[]  SumDenOutMax=[]  SumNumOutMin=[]  SumNumOutMax=[]  DivideOutMin=[]  DivideOutMax=[]  UdiffTsProdOutMin=[]  UdiffTsProdOutMax=[]  NTsProdOutMin=[]  NTsProdOutMax=[]  UintegralTsProdOutMin=[]  UintegralTsProdOutMax=[]  UngainTsProdOutMin=[]  UngainTsProdOutMax=[]  IntegratorContinuousStateAttributes=''  IntegratorStateMustResolveToSignalObject=off  IntegratorRTWStateStorageClass=Auto  FilterContinuousStateAttributes=''  FilterStateMustResolveToSignalObject=off  FilterRTWStateStorageClass=Auto  ParallelPVariant=InternalParameters  IdealPVariant=Disabled  IVariant=InternalParameters  DVariant=Disabled  IntegratorVariant=Continuous  SatVariant=Disabled  AWVariant=Passthrough  PCopyVariant=Disabled  TRVariant=Disabled  FdbkBlocksVariant=Forward  IdealPFdbkVariant=Disabled  SatFdbkVariant=Disabled  DerivativeFilterVariant=Disabled  NVariant=Disabled  NCopyVariant=Disabled_SignalSpec  FilterICVariant=Disabled  IntegratorICVariant=InternalICs  ExternalResetVariant=Disabled  TRSumVariant=Passthrough  SumFdbkVariant=Disabled  SumVariant=Sum_PI  TsampFilterVariant=InternalTs  TsampNgainVariant=Passthrough  TsampIntegralVariant=Passthrough  ExternalSaturationOutDataTypeStr=Inherit: Same as second input
  PID Controller3 : pid_lib/PID Controller  Controller=PI  Form=Parallel  TimeDomain=Continuous-time  UseExternalTs=off  SampleTime=-1  IntegratorMethod=Forward Euler  FilterMethod=Forward Euler  ControllerParametersSource=internal  P=C_pi.Kp  I=C_pi.Ki  D=0  UseFilter=on  N=100  TunerSelectOption=Frequency Response Based  InitialConditionSource=internal  InitialConditionForIntegrator=0  InitialConditionForFilter=0  DifferentiatorICPrevScaledInput=0  ExternalReset=none  TrackingMode=off  Kt=1  LimitOutput=off  SatLimitsSource=internal  UpperSaturationLimit=0.95  LowerSaturationLimit=0.275  LinearizeAsGain=on  AntiWindupMode=none  Kb=1  POutMin=[]  POutMax=[]  IOutMin=[]  IOutMax=[]  DOutMin=[]  DOutMax=[]  NOutMin=[]  NOutMax=[]  SumOutMin=[]  SumOutMax=[]  SaturationOutMin=[]  SaturationOutMax=[]  PParamMin=[]  PParamMax=[]  IParamMin=[]  IParamMax=[]  DParamMin=[]  DParamMax=[]  NParamMin=[]  NParamMax=[]  KbParamMin=[]  KbParamMax=[]  KtParamMin=[]  KtParamMax=[]  KbOutMin=[]  KbOutMax=[]  KtOutMin=[]  KtOutMax=[]  IntegratorOutMin=[]  IntegratorOutMax=[]  FilterOutMin=[]  FilterOutMax=[]  SumI1OutMin=[]  SumI1OutMax=[]  SumI2OutMin=[]  SumI2OutMax=[]  SumI3OutMin=[]  SumI3OutMax=[]  SumI4OutMin=[]  SumI4OutMax=[]  SumDOutMin=[]  SumDOutMax=[]  DifferentiatorOutMin=[]  DifferentiatorOutMax=[]  FilterDiffOutCoefMin=[]  FilterDiffOutCoefMax=[]  ReciprocalOutMin=[]  ReciprocalOutMax=[]  SumDenOutMin=[]  SumDenOutMax=[]  SumNumOutMin=[]  SumNumOutMax=[]  DivideOutMin=[]  DivideOutMax=[]  UdiffTsProdOutMin=[]  UdiffTsProdOutMax=[]  NTsProdOutMin=[]  NTsProdOutMax=[]  UintegralTsProdOutMin=[]  UintegralTsProdOutMax=[]  UngainTsProdOutMin=[]  UngainTsProdOutMax=[]  IntegratorContinuousStateAttributes=''  IntegratorStateMustResolveToSignalObject=off  IntegratorRTWStateStorageClass=Auto  FilterContinuousStateAttributes=''  FilterStateMustResolveToSignalObject=off  FilterRTWStateStorageClass=Auto  ParallelPVariant=InternalParameters  IdealPVariant=Disabled  IVariant=InternalParameters  DVariant=Disabled  IntegratorVariant=Continuous  SatVariant=Disabled  AWVariant=Passthrough  PCopyVariant=Disabled  TRVariant=Disabled  FdbkBlocksVariant=Forward  IdealPFdbkVariant=Disabled  SatFdbkVariant=Disabled  DerivativeFilterVariant=Disabled  NVariant=Disabled  NCopyVariant=Disabled_SignalSpec  FilterICVariant=Disabled  IntegratorICVariant=InternalICs  ExternalResetVariant=Disabled  TRSumVariant=Passthrough  SumFdbkVariant=Disabled  SumVariant=Sum_PI  TsampFilterVariant=InternalTs  TsampNgainVariant=Passthrough  TsampIntegralVariant=Passthrough  ExternalSaturationOutDataTypeStr=Inherit: Same as second input
  PID Controller4 : pid_lib/PID Controller  Controller=PI  Form=Parallel  TimeDomain=Continuous-time  UseExternalTs=off  SampleTime=-1  IntegratorMethod=Forward Euler  FilterMethod=Forward Euler  ControllerParametersSource=internal  P=C_pi.Kp  I=C_pi.Ki  D=0  UseFilter=on  N=100  TunerSelectOption=Frequency Response Based  InitialConditionSource=internal  InitialConditionForIntegrator=0  InitialConditionForFilter=0  DifferentiatorICPrevScaledInput=0  ExternalReset=none  TrackingMode=off  Kt=1  LimitOutput=off  SatLimitsSource=internal  UpperSaturationLimit=0.95  LowerSaturationLimit=0.275  LinearizeAsGain=on  AntiWindupMode=none  Kb=1  POutMin=[]  POutMax=[]  IOutMin=[]  IOutMax=[]  DOutMin=[]  DOutMax=[]  NOutMin=[]  NOutMax=[]  SumOutMin=[]  SumOutMax=[]  SaturationOutMin=[]  SaturationOutMax=[]  PParamMin=[]  PParamMax=[]  IParamMin=[]  IParamMax=[]  DParamMin=[]  DParamMax=[]  NParamMin=[]  NParamMax=[]  KbParamMin=[]  KbParamMax=[]  KtParamMin=[]  KtParamMax=[]  KbOutMin=[]  KbOutMax=[]  KtOutMin=[]  KtOutMax=[]  IntegratorOutMin=[]  IntegratorOutMax=[]  FilterOutMin=[]  FilterOutMax=[]  SumI1OutMin=[]  SumI1OutMax=[]  SumI2OutMin=[]  SumI2OutMax=[]  SumI3OutMin=[]  SumI3OutMax=[]  SumI4OutMin=[]  SumI4OutMax=[]  SumDOutMin=[]  SumDOutMax=[]  DifferentiatorOutMin=[]  DifferentiatorOutMax=[]  FilterDiffOutCoefMin=[]  FilterDiffOutCoefMax=[]  ReciprocalOutMin=[]  ReciprocalOutMax=[]  SumDenOutMin=[]  SumDenOutMax=[]  SumNumOutMin=[]  SumNumOutMax=[]  DivideOutMin=[]  DivideOutMax=[]  UdiffTsProdOutMin=[]  UdiffTsProdOutMax=[]  NTsProdOutMin=[]  NTsProdOutMax=[]  UintegralTsProdOutMin=[]  UintegralTsProdOutMax=[]  UngainTsProdOutMin=[]  UngainTsProdOutMax=[]  IntegratorContinuousStateAttributes=''  IntegratorStateMustResolveToSignalObject=off  IntegratorRTWStateStorageClass=Auto  FilterContinuousStateAttributes=''  FilterStateMustResolveToSignalObject=off  FilterRTWStateStorageClass=Auto  ParallelPVariant=InternalParameters  IdealPVariant=Disabled  IVariant=InternalParameters  DVariant=Disabled  IntegratorVariant=Continuous  SatVariant=Disabled  AWVariant=Passthrough  PCopyVariant=Disabled  TRVariant=Disabled  FdbkBlocksVariant=Forward  IdealPFdbkVariant=Disabled  SatFdbkVariant=Disabled  DerivativeFilterVariant=Disabled  NVariant=Disabled  NCopyVariant=Disabled_SignalSpec  FilterICVariant=Disabled  IntegratorICVariant=InternalICs  ExternalResetVariant=Disabled  TRSumVariant=Passthrough  SumFdbkVariant=Disabled  SumVariant=Sum_PI  TsampFilterVariant=InternalTs  TsampNgainVariant=Passthrough  TsampIntegralVariant=Passthrough  ExternalSaturationOutDataTypeStr=Inherit: Same as second input
  Product : Product
  Product1 : Product
  Sum{1,4,7..8} (4 alike) : Sum  Inputs=|+-
  Sum5 : Sum  Inputs=|+++
  Sum6 : Sum  Inputs=|-++
  dq0 to Alpha-Beta-Zero : powerlib_meascontrol/Transformations/dq0 to Alpha-Beta-Zero  Alignment=90 degrees behind phase A axis
      settings: SourceProductBaseCode=PS
  Uref : Outport
  wires:
  Sum1/1 -> PID Controller1/1
  Vq/1 -> Sum6/3, Sum4/2
  Mux1/1 -> dq0 to Alpha-Beta-Zero/1
  [Ed] -> Mux1/1
  Sum4/1 -> PID Controller2/1
  Vd/1 -> Sum5/3, Sum1/2
  Apparent Voltage Ref/1 -> Sum4/1
  [Eq] -> Mux1/2
  Real Voltage Ref/1 -> Sum1/1
  PID Controller1/1 -> Product1/2, Sum7/1
  PID Controller2/1 -> Product/2, Sum8/1
  PID Controller4/1 -> Sum6/2
  wt/1 -> dq0 to Alpha-Beta-Zero/2
  dq0 to Alpha-Beta-Zero/1 -> Uref/1
  [w] -> Gain/1
  PID Controller3/1 -> Sum5/1
  Sum5/1 -> [Ed]
  Product/1 -> Sum5/2
  Sum6/1 -> [Eq]
  Gain/1 -> Product1/1, Product/1
  Product1/1 -> Sum6/1
  w/1 -> [w]
  Sum7/1 -> PID Controller3/1
  Id/1 -> Sum7/2
  Sum8/1 -> PID Controller4/1
  Iq/1 -> Sum8/2

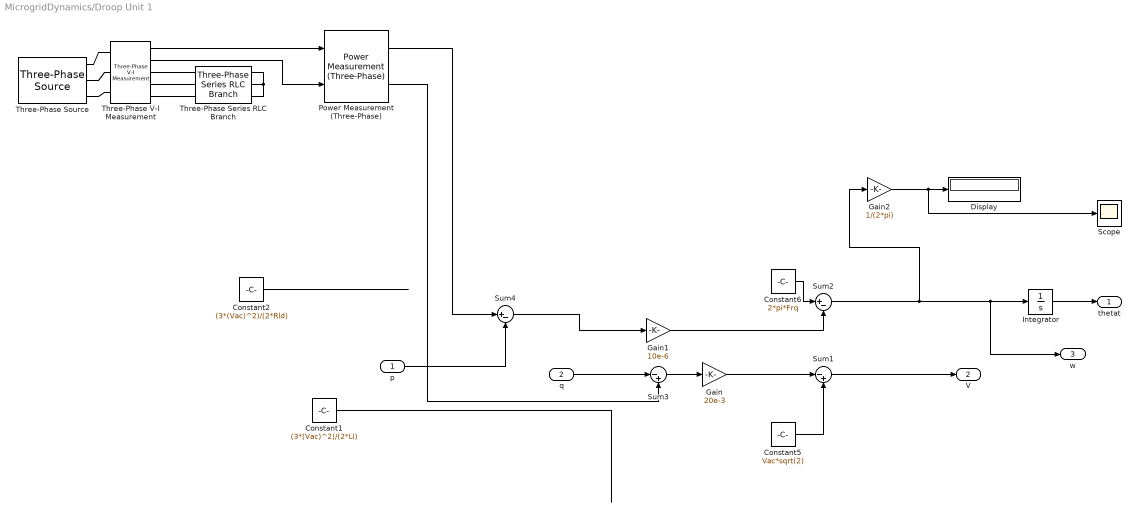
== system MicrogridDynamics/Droop Unit 1 ==
  p : Inport
  q : Inport  Port=2
  Constant1 : Constant  Value=(3*(Vac)^2)/(2*Ll)
  Constant2 : Constant  Value=(3*(Vac)^2)/(2*Rld)
  Constant5 : Constant  Value=Vac*sqrt(2)
  Constant6 : Constant  Value=2*pi*Frq
  Display : Display
  Gain : Gain  Gain=20e-3
  Gain1 : Gain  Gain=10e-6
  Gain2 : Gain  Gain=1/(2*pi)
  Integrator : Integrator
  Power Measurement (Three-Phase) : eePowerMeasurement/Power Measurement (Three-Phase)  LabelModeActiveChoice=Continuous  F=50  K=[0]  Seq=Positive  Ts=0
      settings: SourceProductBaseCode=PS
  Scope : Scope
  Sum1 : Sum  Inputs=|-+
  Sum2 : Sum  Inputs=|+-
  Sum3 : Sum  Inputs=|-+
  Sum4 : Sum  Inputs=|+-
  Three-Phase Series RLC Branch : powerlib/Elements/Three-Phase Series RLC Branch  LConnTagsString=A|B|C  RConnTagsString=A|B|C  BranchType=R  Resistance=50  Inductance=1e-3  Capacitance=1e-6  Measurements=None
  Three-Phase V-I Measurement : powerlib/Measurements/Three-Phase V-I Measurement  VoltageMeasurement=phase-to-ground  SetLabelV=off  LabelV=Vabc  Vpu=off  VpuLL=off  CurrentMeasurement=yes  SetLabelI=off  LabelI=Iabc  Ipu=off  Pbase=100e6  Vbase=500e3  OutputType=Complex  PhasorSimulation=off  PSBequivalent=0
  Three-Phase Source : powerlib/Electrical Sources/Three-Phase Source  InternalConnection=Yg  VoltagePhases=off  Voltage=Vac  PhaseAngle=0  Voltage_phases=[25e3 25e3 25e3]/sqrt(3)  PhaseAngles_phases=[0 -120 +120]  Frequency=50  NonIdealSource=on  SpecifyImpedance=off  Resistance=0.01  Inductance=16.58e-3  ShortCircuitLevel=100e6  BaseVoltage=Vac  XRratio=7  BusType=swing  Pref=10e3  Qref=0  Prefabc=[10e3, 10e3, 10e3]  Qrefabc=[0, 0, 0]  Qmin=-inf  Qmax=inf
  thetat : Outport
  V : Outport  Port=2
  w : Outport  Port=3
  wires:
  Constant5/1 -> Sum1/2
  Constant6/1 -> Sum2/1
  q/1 -> Sum3/1
  Integrator/1 -> thetat/1
  Sum3/1 -> Gain/1
  Gain2/1 -> Scope/1, Display/1
  Sum2/1 -> Gain2/1, w/1, Integrator/1
  Sum1/1 -> V/1
  Gain/1 -> Sum1/1
  Gain1/1 -> Sum2/2
  p/1 -> Sum4/2
  Constant1/1 -> ?
  Constant2/1 -> ?
  Sum4/1 -> Gain1/1
  Three-Phase V-I Measurement/1 -> Power Measurement (Three-Phase)/1
  Three-Phase V-I Measurement/2 -> Power Measurement (Three-Phase)/2
  Power Measurement (Three-Phase)/1 -> Sum4/1
  Power Measurement (Three-Phase)/2 -> Sum3/2
  connections:
  Three-Phase V-I Measurement/LConn1 -- Three-Phase Source/RConn1
  Three-Phase Source/RConn2 -- Three-Phase V-I Measurement/LConn2
  Three-Phase Source/RConn3 -- Three-Phase V-I Measurement/LConn3
  Three-Phase Series RLC Branch/LConn1 -- Three-Phase V-I Measurement/RConn1
  Three-Phase V-I Measurement/RConn2 -- Three-Phase Series RLC Branch/LConn2
  Three-Phase V-I Measurement/RConn3 -- Three-Phase Series RLC Branch/LConn3
  Three-Phase Series RLC Branch/RConn1 -- Three-Phase Series RLC Branch/RConn2 -- Three-Phase Series RLC Branch/RConn3

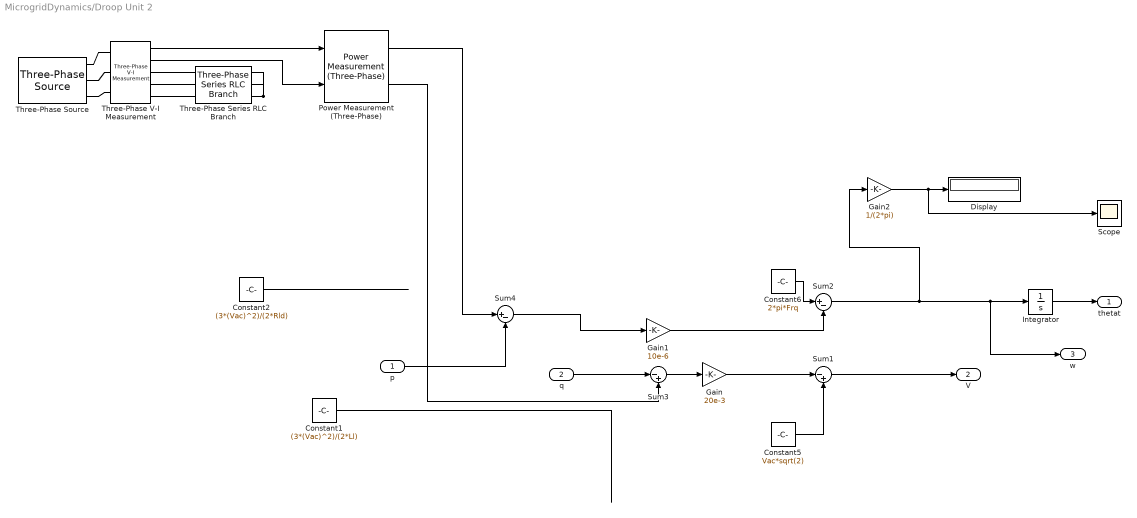
== system MicrogridDynamics/Droop Unit 2 ==
  p : Inport
  q : Inport  Port=2
  Constant1 : Constant  Value=(3*(Vac)^2)/(2*Ll)
  Constant2 : Constant  Value=(3*(Vac)^2)/(2*Rld)
  Constant5 : Constant  Value=Vac*sqrt(2)
  Constant6 : Constant  Value=2*pi*Frq
  Display : Display
  Gain : Gain  Gain=20e-3
  Gain1 : Gain  Gain=10e-6
  Gain2 : Gain  Gain=1/(2*pi)
  Integrator : Integrator
  Power Measurement (Three-Phase) : eePowerMeasurement/Power Measurement (Three-Phase)  LabelModeActiveChoice=Continuous  F=50  K=[0]  Seq=Positive  Ts=0
      settings: SourceProductBaseCode=PS
  Scope : Scope
  Sum1 : Sum  Inputs=|-+
  Sum2 : Sum  Inputs=|+-
  Sum3 : Sum  Inputs=|-+
  Sum4 : Sum  Inputs=|+-
  Three-Phase Series RLC Branch : powerlib/Elements/Three-Phase Series RLC Branch  LConnTagsString=A|B|C  RConnTagsString=A|B|C  BranchType=R  Resistance=50  Inductance=1e-3  Capacitance=1e-6  Measurements=None
  Three-Phase V-I Measurement : powerlib/Measurements/Three-Phase V-I Measurement  VoltageMeasurement=phase-to-ground  SetLabelV=off  LabelV=Vabc  Vpu=off  VpuLL=off  CurrentMeasurement=yes  SetLabelI=off  LabelI=Iabc  Ipu=off  Pbase=100e6  Vbase=500e3  OutputType=Complex  PhasorSimulation=off  PSBequivalent=0
  Three-Phase Source : powerlib/Electrical Sources/Three-Phase Source  InternalConnection=Yg  VoltagePhases=off  Voltage=Vac  PhaseAngle=0  Voltage_phases=[25e3 25e3 25e3]/sqrt(3)  PhaseAngles_phases=[0 -120 +120]  Frequency=50  NonIdealSource=on  SpecifyImpedance=off  Resistance=0.01  Inductance=16.58e-3  ShortCircuitLevel=100e6  BaseVoltage=Vac  XRratio=7  BusType=swing  Pref=10e3  Qref=0  Prefabc=[10e3, 10e3, 10e3]  Qrefabc=[0, 0, 0]  Qmin=-inf  Qmax=inf
  thetat : Outport
  V : Outport  Port=2
  w : Outport  Port=3
  wires:
  Constant5/1 -> Sum1/2
  Constant6/1 -> Sum2/1
  q/1 -> Sum3/1
  Integrator/1 -> thetat/1
  Sum3/1 -> Gain/1
  Gain2/1 -> Scope/1, Display/1
  Sum2/1 -> Gain2/1, w/1, Integrator/1
  Sum1/1 -> V/1
  Gain/1 -> Sum1/1
  Gain1/1 -> Sum2/2
  p/1 -> Sum4/2
  Constant1/1 -> ?
  Constant2/1 -> ?
  Sum4/1 -> Gain1/1
  Three-Phase V-I Measurement/1 -> Power Measurement (Three-Phase)/1
  Three-Phase V-I Measurement/2 -> Power Measurement (Three-Phase)/2
  Power Measurement (Three-Phase)/1 -> Sum4/1
  Power Measurement (Three-Phase)/2 -> Sum3/2
  connections:
  Three-Phase V-I Measurement/LConn1 -- Three-Phase Source/RConn1
  Three-Phase Source/RConn2 -- Three-Phase V-I Measurement/LConn2
  Three-Phase Source/RConn3 -- Three-Phase V-I Measurement/LConn3
  Three-Phase Series RLC Branch/LConn1 -- Three-Phase V-I Measurement/RConn1
  Three-Phase V-I Measurement/RConn2 -- Three-Phase Series RLC Branch/LConn2
  Three-Phase V-I Measurement/RConn3 -- Three-Phase Series RLC Branch/LConn3
  Three-Phase Series RLC Branch/RConn3 -- Three-Phase Series RLC Branch/RConn1 -- Three-Phase Series RLC Branch/RConn2

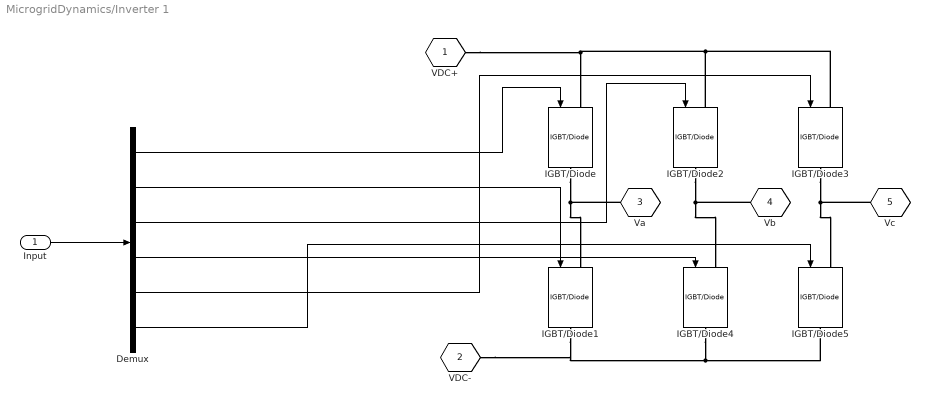
== system MicrogridDynamics/Inverter 1 ==
  Input : Inport
  Demux : Demux  Outputs=6
  IGBT/Diode{,1..5} (6 alike) : powerlib/Power Electronics/IGBT//Diode  Ron=1e-3  Rs=1e5  Cs=inf  Measurements=off
  VDC+ : PMIOPort  Tag=PMCPort  Side=Left
  VDC- : PMIOPort  Tag=PMCPort  Port=2  Side=Left
  Va : PMIOPort  Tag=PMCPort  Port=3  Side=Right
  Vb : PMIOPort  Tag=PMCPort  Port=4  Side=Right
  Vc : PMIOPort  Tag=PMCPort  Port=5  Side=Right
  wires:
  Demux/6 -> IGBT/Diode5/1
  Demux/5 -> IGBT/Diode3/1
  Demux/3 -> IGBT/Diode2/1
  Demux/1 -> IGBT/Diode/1
  Demux/4 -> IGBT/Diode4/1
  Demux/2 -> IGBT/Diode1/1
  Input/1 -> Demux/1
  connections:
  IGBT/Diode2/RConn1 -- IGBT/Diode4/LConn1 -- Vb/RConn1
  IGBT/Diode4/RConn1 -- IGBT/Diode5/RConn1 -- VDC-/RConn1 -- IGBT/Diode1/RConn1
  IGBT/Diode3/RConn1 -- IGBT/Diode5/LConn1 -- Vc/RConn1
  IGBT/Diode2/LConn1 -- IGBT/Diode3/LConn1 -- VDC+/RConn1 -- IGBT/Diode/LConn1
  IGBT/Diode/RConn1 -- IGBT/Diode1/LConn1 -- Va/RConn1

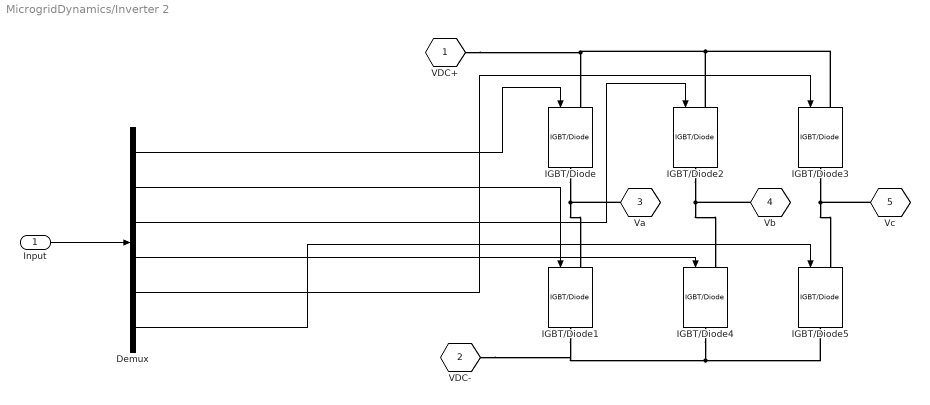
== system MicrogridDynamics/Inverter 2 ==
  Input : Inport
  Demux : Demux  Outputs=6
  IGBT/Diode{,1..5} (6 alike) : powerlib/Power Electronics/IGBT//Diode  Ron=1e-3  Rs=1e5  Cs=inf  Measurements=off
  VDC+ : PMIOPort  Tag=PMCPort  Side=Left
  VDC- : PMIOPort  Tag=PMCPort  Port=2  Side=Left
  Va : PMIOPort  Tag=PMCPort  Port=3  Side=Right
  Vb : PMIOPort  Tag=PMCPort  Port=4  Side=Right
  Vc : PMIOPort  Tag=PMCPort  Port=5  Side=Right
  wires:
  Demux/6 -> IGBT/Diode5/1
  Demux/5 -> IGBT/Diode3/1
  Demux/3 -> IGBT/Diode2/1
  Demux/1 -> IGBT/Diode/1
  Demux/4 -> IGBT/Diode4/1
  Demux/2 -> IGBT/Diode1/1
  Input/1 -> Demux/1
  connections:
  IGBT/Diode2/RConn1 -- IGBT/Diode4/LConn1 -- Vb/RConn1
  IGBT/Diode4/RConn1 -- IGBT/Diode5/RConn1 -- VDC-/RConn1 -- IGBT/Diode1/RConn1
  IGBT/Diode3/RConn1 -- IGBT/Diode5/LConn1 -- Vc/RConn1
  IGBT/Diode2/LConn1 -- IGBT/Diode3/LConn1 -- IGBT/Diode/LConn1 -- VDC+/RConn1
  IGBT/Diode/RConn1 -- IGBT/Diode1/LConn1 -- Va/RConn1

== system MicrogridDynamics/PWM generator1 ==
  Vref : Inport
  Demux : Demux  Outputs=3
  SVPWM Generator (2-Level)3 : powerlib_meascontrol/Pulse & Signal Generators/SVPWM Generator (2-Level)  InputType=alpha-beta components  SwitchingPattern=Pattern #1  Fc=10e3  ParUref=[0.8 -30 50]  Ts=0
      settings: SourceProductBaseCode=PS
  Scope : Scope
  PWM : Outport
  wires:
  Vref/1 -> Demux/1
  Demux/3 -> ?
  SVPWM Generator (2-Level)3/1 -> PWM/1
  Demux/2 -> SVPWM Generator (2-Level)3/2
  Demux/1 -> SVPWM Generator (2-Level)3/1, Scope/1

== system MicrogridDynamics/PWM generator2 ==
  Vref : Inport
  Demux : Demux  Outputs=3
  SVPWM Generator (2-Level)3 : powerlib_meascontrol/Pulse & Signal Generators/SVPWM Generator (2-Level)  InputType=alpha-beta components  SwitchingPattern=Pattern #1  Fc=10e3  ParUref=[0.8 -30 50]  Ts=0
      settings: SourceProductBaseCode=PS
  Scope : Scope
  PWM : Outport
  wires:
  Vref/1 -> Demux/1
  Demux/3 -> ?
  SVPWM Generator (2-Level)3/1 -> PWM/1
  Demux/2 -> SVPWM Generator (2-Level)3/2
  Demux/1 -> SVPWM Generator (2-Level)3/1, Scope/1

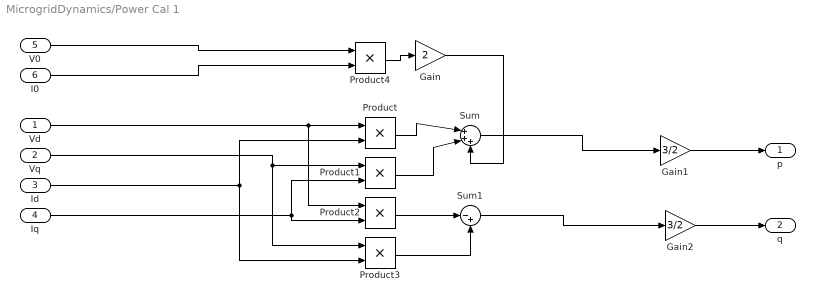
== system MicrogridDynamics/Power Cal 1 ==
  Vd : Inport
  Vq : Inport  Port=2
  Id : Inport  Port=3
  Iq : Inport  Port=4
  V0 : Inport  Port=5
  I0 : Inport  Port=6
  Gain : Gain  Gain=2
  Gain1 : Gain  Gain=3/2
  Gain2 : Gain  Gain=3/2
  Product{,1..4} (5 alike) : Product
  Sum : Sum  Inputs=|+++
  Sum1 : Sum  Inputs=|-+
  p : Outport
  q : Outport  Port=2
  wires:
  Sum1/1 -> Gain2/1
  Product/1 -> Sum/1
  Id/1 -> Product/2, Product3/2
  Product1/1 -> Sum/2
  Product2/1 -> Sum1/1
  Vd/1 -> Product2/1, Product/1
  Sum/1 -> Gain1/1
  Product3/1 -> Sum1/2
  Vq/1 -> Product3/1, Product1/1
  Iq/1 -> Product1/2, Product2/2
  V0/1 -> Product4/1
  I0/1 -> Product4/2
  Product4/1 -> Gain/1
  Gain/1 -> Sum/3
  Gain1/1 -> p/1
  Gain2/1 -> q/1
